simulink library "INT_InjCrv_PiI1Set"  (R2016b)
settings: Solver=VariableStepAuto  StartTime=0.0  StopTime=10.0  RelTol=1e-3
settings Model: Creator=mayongchao  LastModifiedBy=mayongchao

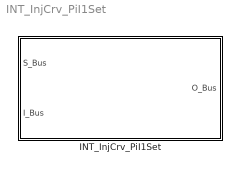
== system INT_InjCrv_PiI1Set ==
  INT_InjCrv_PiI1Set : Subsystem

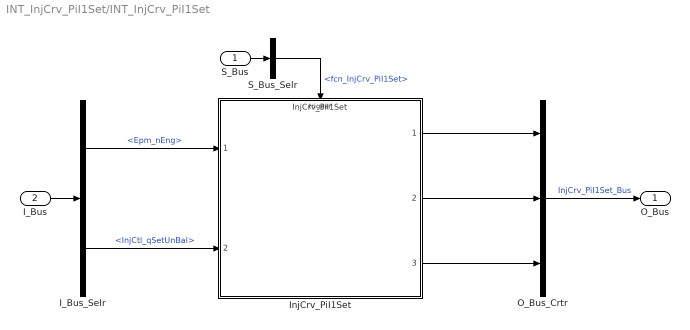
== system INT_InjCrv_PiI1Set/INT_InjCrv_PiI1Set ==
  S_Bus : Inport
  I_Bus : Inport  Port=2
  I_Bus_Selr : BusSelector  OutputSignals=Epm_nEng,InjCtl_qSetUnBal
  InjCrv_PiI1Set : ModelReference  ModelNameDialog=InjCrv_PiI1Set  SimulationMode=Normal  ModelReferenceVersion=1.15  TriggerPortName=function  TriggerPortTriggerType=function-call  TriggerPortStatesWhenEnabling=held
  O_Bus_Crtr : BusCreator  Inputs=3
  S_Bus_Selr : BusSelector  OutputSignals=fcn_InjCrv_PiI1Set
  O_Bus : Outport
  wires:
  S_Bus_Selr/1 -> InjCrv_PiI1Set/Trigger  "<fcn_InjCrv_PiI1Set>"
  S_Bus/1 -> S_Bus_Selr/1
  I_Bus/1 -> I_Bus_Selr/1
  I_Bus_Selr/1 -> InjCrv_PiI1Set/1  "<Epm_nEng>"
  I_Bus_Selr/2 -> InjCrv_PiI1Set/2  "<InjCtl_qSetUnBal>"
  O_Bus_Crtr/1 -> O_Bus/1  "InjCrv_PiI1Set_Bus"
  InjCrv_PiI1Set/1 -> O_Bus_Crtr/1
  InjCrv_PiI1Set/2 -> O_Bus_Crtr/2
  InjCrv_PiI1Set/3 -> O_Bus_Crtr/3
